simulink model "B3333"  (R2016a)
settings: Solver=FixedStepDiscrete  StartTime=0.0  StopTime=inf  RelTol=1e-3
undefined symbols (not defined in the file): DiscIntNeverNeededParam, Green, led0, Rec, SDTV
libraries: embdlinuxlib x13, visionconversions x8
settings Model: SimulationMode=external  ExtModeTrigDuration=100  Creator=The MathWorks, Inc.  LastModifiedBy=Yewly
settings SolverCC: PositivePriorityOrder=on
settings DataIOCC: LimitDataPoints=on  SaveFormat=Array
settings OptimizationCC: ExpressionDepthLimit=2147483647  OptimizeModelRefInitCode=on  LifeSpan=Inf  MaxStackSize=64
settings DebuggingCC: UnderspecifiedInitializationDetection=Classic  MergeDetectMultiDrivingBlocksExec=none  MultiTaskRateTransMsg=warning  FcnCallInpInsideContextMsg=EnableAllAsWarning  AllowSymbolicDim=off  StateNameClashWarn=warning
settings HardwareCC: ProdBitPerPointer=32  ProdLargestAtomicInteger=Long  ProdLargestAtomicFloat=Double  ProdWordSize=32  ProdHWDeviceType=ARM Compatible->ARM Cortex  UseEmbeddedCoderFeatures=off  UseSimulinkCoderFeatures=off
settings ModelReferenceCC: PropagateSignalLabelsOutOfModel=off
settings RTWCC: SystemTargetFile=ert.tlc  HardwareBoard=Raspberry Pi  TemplateMakefile=ert_default_tmf  GenerateReport=on  RTWVerbose=off  Toolchain=GNU GCC Raspberry Pi  LaunchReport=on
settings CodeAppCC: ForceParamTrailComments=on  IgnoreCustomStorageClasses=off  OperatorAnnotations=on  SimulinkDataObjDesc=on  SFDataObjDesc=on  MATLABFcnDesc=on  MangleLength=10  CustomSymbolStrType=$N$R$M  InsertBlockDesc=on  MATLABSourceComments=on  InternalIdentifier=Classic
settings ERTTargetCC: SupportNonInlinedSFcns=on
settings ConfigComp: CovModelRefEnable=Off

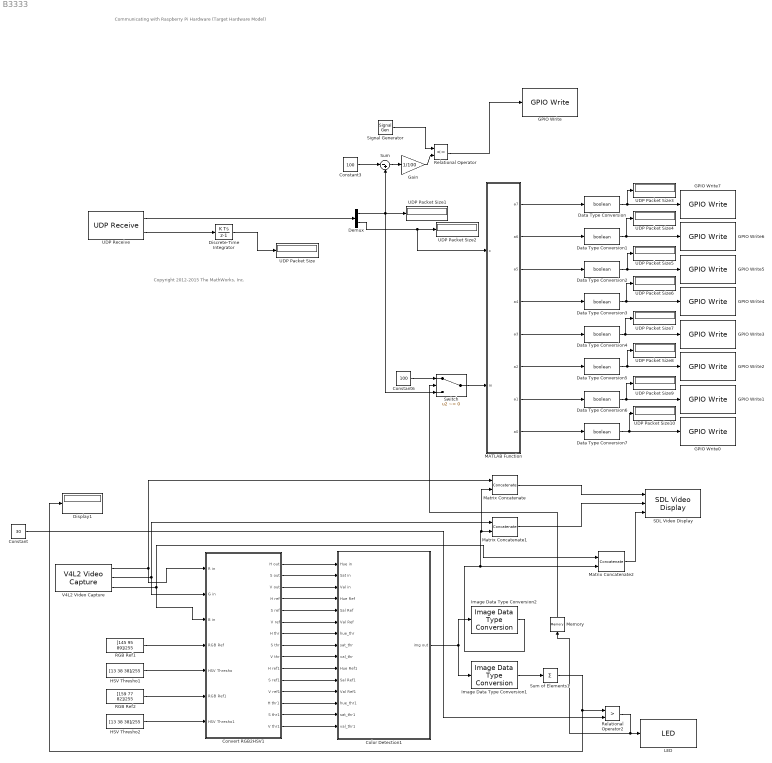
== system B3333 ==
  note: Communicating with Raspberry Pi Hardware
      | (Target Hardware Model)
  note: Copyright 2012-2015 The MathWorks, Inc.
  Color Detection1 : Subsystem
  Constant : Constant  Value=30
  Constant3 : Constant  Value=100
  Constant6 : Constant  Value=100
  Convert RGB2HSV1 : Subsystem
  Data Type Conversion{,1..7} (8 alike) : DataTypeConversion  OutDataTypeStr=boolean
  Demux : Demux  Outputs=2
  Discrete-Time Integrator : DiscreteIntegrator  gainval=1e4  SampleTime=-1  ICPrevOutput=DiscIntNeverNeededParam  ICPrevScaledInput=DiscIntNeverNeededParam
  Display1 : Display
  GPIO Write : embdlinuxlib/GPIO Write  board=Pi 3 Model B  gpio=17  direction=Output  blockPlatform=Raspberry Pi
  GPIO Write0 : embdlinuxlib/GPIO Write  board=Pi 3 Model B  gpio=18  direction=Output  blockPlatform=Raspberry Pi
  GPIO Write1 : embdlinuxlib/GPIO Write  board=Pi 3 Model B  gpio=23  direction=Output  blockPlatform=Raspberry Pi
  GPIO Write2 : embdlinuxlib/GPIO Write  board=Pi 3 Model B  gpio=24  direction=Output  blockPlatform=Raspberry Pi
  GPIO Write3 : embdlinuxlib/GPIO Write  board=Pi 3 Model B  gpio=25  direction=Output  blockPlatform=Raspberry Pi
  GPIO Write4 : embdlinuxlib/GPIO Write  board=Pi 3 Model B  gpio=8  direction=Output  blockPlatform=Raspberry Pi
  GPIO Write5 : embdlinuxlib/GPIO Write  board=Pi 3 Model B  gpio=7  direction=Output  blockPlatform=Raspberry Pi
  GPIO Write6 : embdlinuxlib/GPIO Write  board=Pi 3 Model B  gpio=12  direction=Output  blockPlatform=Raspberry Pi
  "GPIO Write7 " : embdlinuxlib/GPIO Write  board=Pi 3 Model B  gpio=16  direction=Output  blockPlatform=Raspberry Pi
  Gain : Gain  Gain=1/100
  HSV Thresho1 : Constant  Value=[13 38 38]/255
  HSV Thresho2 : Constant  Value=[13 38 38]/255
  Image Data Type Conversion1 : visionconversions/Image Data Type Conversion  outDT=double  isSigned=on  wordLen=16  numFracBits=0
  Image Data Type Conversion2 : visionconversions/Image Data Type Conversion  outDT=uint8  isSigned=on  wordLen=16  numFracBits=0
  LED : embdlinuxlib/LED  board=Model B+  led=led0 (Green)  blockPlatform=Raspberry Pi
  MATLAB Function : MATLAB Function  TreatAsAtomicUnit=on
  Matrix Concatenate : Concatenate  Mode=Multidimensional array  ConcatenateDimension=2
  Matrix Concatenate1 : Concatenate  Mode=Multidimensional array  ConcatenateDimension=2
  Matrix Concatenate2 : Concatenate  Mode=Multidimensional array  ConcatenateDimension=2
  Memory : Memory
  RGB Ref1 : Constant  Value=[145 95 89]/255
  RGB Ref2 : Constant  Value=[159 77 82]/255
  Relational Operator : RelationalOperator  Operator=<=  OutDataTypeStr=boolean
  Relational Operator2 : RelationalOperator  Operator=>  OutDataTypeStr=boolean
  SDL Video Display : embdlinuxlib/SDL Video Display  pixelFormat=RGB  pixelOrder=Planar  rowMajor=on  blockPlatform=Raspberry Pi
  Signal Generator : SignalGenerator  WaveForm=sawtooth  Frequency=200
  Sum : Sum  Inputs=|-+
  Sum of Elements1 : Sum  Inputs=+
  Switch : Switch  Criteria=u2 ~= 0  Threshold=250
  UDP Packet Size{,1..10} (11 alike) : Display
  UDP Receive : embdlinuxlib/UDP Receive  localURL='0.0.0.0'  localPort=25001  remoteURL='0.0.0.0'  remotePort=-1  recvBufferSize=8192  signalDatatype=uint8  dims=2  isVarSize=off  showBlockingTime=off  blockingTime=0  sampletime=1/10000  blockPlatform=Raspberry Pi
  V4L2 Video Capture : embdlinuxlib/V4L2 Video Capture  m_devName='/dev/video0'  roi=[0, 0, 640, 480]  imSizeSelection=Custom  imSize=[80 60]  pixelFormat=RGB  pixelOrder=Planar  sampleTime=1/50  simOutput=Colorbars  blockPlatform=Raspberry Pi
  wires:
  UDP Receive/2 -> Discrete-Time Integrator/1
  Discrete-Time Integrator/1 -> UDP Packet Size/1
  UDP Receive/1 -> Demux/1
  Relational Operator/1 -> GPIO Write/1
  Signal Generator/1 -> Relational Operator/1
  Demux/1 -> Switch/3, Sum/2, UDP Packet Size1/1
  Constant3/1 -> Sum/1
  Sum/1 -> Gain/1
  Gain/1 -> Relational Operator/2
  MATLAB Function/1(a7) -> Data Type Conversion/1
  Data Type Conversion/1 -> UDP Packet Size3/1, "GPIO Write7 "/1
  MATLAB Function/2(a6) -> Data Type Conversion1/1
  Data Type Conversion1/1 -> UDP Packet Size4/1, GPIO Write6/1
  MATLAB Function/3(a5) -> Data Type Conversion2/1
  Data Type Conversion2/1 -> UDP Packet Size5/1, GPIO Write5/1
  MATLAB Function/4(a4) -> Data Type Conversion3/1
  Data Type Conversion3/1 -> GPIO Write4/1, UDP Packet Size6/1
  MATLAB Function/5(a3) -> Data Type Conversion4/1
  Data Type Conversion4/1 -> UDP Packet Size7/1, GPIO Write3/1
  MATLAB Function/6(a2) -> Data Type Conversion5/1
  Data Type Conversion5/1 -> UDP Packet Size8/1, GPIO Write2/1
  MATLAB Function/7(a1) -> Data Type Conversion6/1
  Data Type Conversion6/1 -> UDP Packet Size9/1, GPIO Write1/1
  MATLAB Function/8(a0) -> Data Type Conversion7/1
  Data Type Conversion7/1 -> UDP Packet Size10/1, GPIO Write0/1
  Demux/2 -> MATLAB Function/1(x), UDP Packet Size2/1
  Switch/1 -> MATLAB Function/2(m)
  Constant6/1 -> Switch/1
  Constant/1 -> Relational Operator2/2
  Relational Operator2/1 -> Memory/1, LED/1
  Color Detection1/1(img out) -> Image Data Type Conversion1/1, Image Data Type Conversion2/1
  Sum of Elements1/1 -> Relational Operator2/1, Display1/1
  Image Data Type Conversion2/1 -> Matrix Concatenate/2, Matrix Concatenate1/2, Matrix Concatenate2/2
  Image Data Type Conversion1/1 -> Sum of Elements1/1
  HSV Thresho1/1 -> Convert RGB2HSV1/5(HSV Thresho)
  Convert RGB2HSV1/2(S out) -> Color Detection1/2(Sat in)
  Convert RGB2HSV1/9(V thr) -> Color Detection1/9(val_thr)
  Convert RGB2HSV1/6(V ref) -> Color Detection1/6(Val Ref)
  Convert RGB2HSV1/3(V out) -> Color Detection1/3("Val in ")
  Convert RGB2HSV1/8(S thr) -> Color Detection1/8(sat_thr)
  Convert RGB2HSV1/1(H out) -> Color Detection1/1("Hue in ")
  Convert RGB2HSV1/4(H ref) -> Color Detection1/4(Hue Ref)
  Convert RGB2HSV1/5(S ref) -> Color Detection1/5(Sal Ref)
  Convert RGB2HSV1/7(H thr) -> Color Detection1/7(hue_thr)
  V4L2 Video Capture/1 -> Matrix Concatenate/1, Convert RGB2HSV1/1(R in)
  V4L2 Video Capture/2 -> Matrix Concatenate1/1, Convert RGB2HSV1/2(G in)
  V4L2 Video Capture/3 -> Matrix Concatenate2/1, Convert RGB2HSV1/3(B in)
  RGB Ref1/1 -> Convert RGB2HSV1/4(RGB Ref)
  Convert RGB2HSV1/10(H ref1) -> Color Detection1/10(Hue Ref1)
  Convert RGB2HSV1/11(S ref1) -> Color Detection1/11(Sal Ref1)
  Convert RGB2HSV1/12(V ref1) -> Color Detection1/12(Val Ref1)
  Convert RGB2HSV1/13(H thr1) -> Color Detection1/13(hue_thr1)
  Convert RGB2HSV1/14(S thr1) -> Color Detection1/14(sat_thr1)
  Convert RGB2HSV1/15(V thr1) -> Color Detection1/15(val_thr1)
  HSV Thresho2/1 -> Convert RGB2HSV1/7(HSV Thresho1)
  RGB Ref2/1 -> Convert RGB2HSV1/6(RGB Ref1)
  Matrix Concatenate/1 -> SDL Video Display/1
  Matrix Concatenate1/1 -> SDL Video Display/2
  Matrix Concatenate2/1 -> SDL Video Display/3
  Memory/1 -> Switch/2

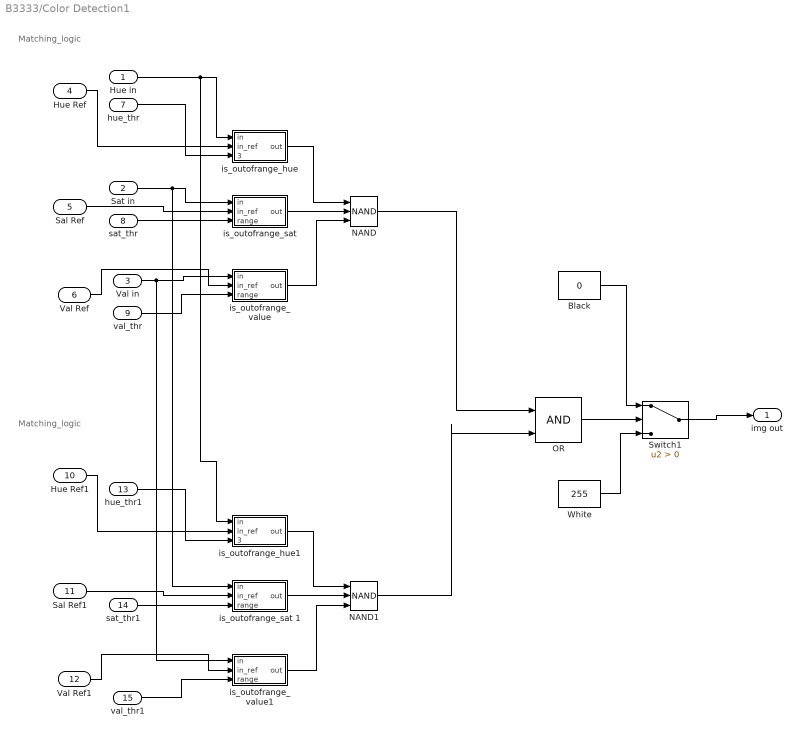
== system B3333/Color Detection1 ==
  note: Matching_logic
  note: Matching_logic
  "Hue in " : Inport
  Sat in : Inport  Port=2
  "Val in " : Inport  Port=3
  Hue Ref : Inport  Port=4
  Sal Ref : Inport  Port=5
  Val Ref : Inport  Port=6
  hue_thr : Inport  Port=7
  sat_thr : Inport  Port=8
  val_thr : Inport  Port=9
  Hue Ref1 : Inport  Port=10
  Sal Ref1 : Inport  Port=11
  Val Ref1 : Inport  Port=12
  hue_thr1 : Inport  Port=13
  sat_thr1 : Inport  Port=14
  val_thr1 : Inport  Port=15
  Black : Constant  Value=0
  NAND : Logic  Operator=NAND  Inputs=3  IconShape=distinctive  AllPortsSameDT=off  OutDataTypeStr=boolean
  NAND1 : Logic  Operator=NAND  Inputs=3  IconShape=distinctive  AllPortsSameDT=off  OutDataTypeStr=boolean
  OR : Logic  IconShape=distinctive  AllPortsSameDT=off  OutDataTypeStr=boolean
  Switch1 : Switch  Criteria=u2 > Threshold  OutDataTypeStr=uint8
  White : Constant  Value=255
  is_outofrange_hue : Subsystem
  is_outofrange_hue1 : Subsystem
  "is_outofrange_sat " : Subsystem
  is_outofrange_sat 1 : Subsystem
  is_outofrange_value : Subsystem
  is_outofrange_value1 : Subsystem
  img out : Outport
  wires:
  is_outofrange_value/1(out) -> NAND/3
  is_outofrange_hue/1(out) -> NAND/1
  Val Ref/1 -> is_outofrange_value/2(in_ref)
  Hue Ref/1 -> is_outofrange_hue/2(in_ref)
  "is_outofrange_sat "/1(out) -> NAND/2
  Sal Ref/1 -> "is_outofrange_sat "/2(in_ref)
  Black/1 -> Switch1/1
  White/1 -> Switch1/3
  hue_thr/1 -> is_outofrange_hue/3("threshold ")
  sat_thr/1 -> "is_outofrange_sat "/3("range ")
  val_thr/1 -> is_outofrange_value/3("range ")
  Switch1/1 -> img out/1
  is_outofrange_value1/1(out) -> NAND1/3
  is_outofrange_hue1/1(out) -> NAND1/1
  "Val in "/1 -> is_outofrange_value1/1(in), is_outofrange_value/1(in)
  Val Ref1/1 -> is_outofrange_value1/2(in_ref)
  Hue Ref1/1 -> is_outofrange_hue1/2(in_ref)
  "Hue in "/1 -> is_outofrange_hue1/1(in), is_outofrange_hue/1(in)
  is_outofrange_sat 1/1(out) -> NAND1/2
  Sal Ref1/1 -> is_outofrange_sat 1/2(in_ref)
  Sat in/1 -> "is_outofrange_sat "/1(in), is_outofrange_sat 1/1(in)
  NAND1/1 -> OR/2
  hue_thr1/1 -> is_outofrange_hue1/3("threshold ")
  sat_thr1/1 -> is_outofrange_sat 1/3("range ")
  val_thr1/1 -> is_outofrange_value1/3("range ")
  NAND/1 -> OR/1
  OR/1 -> Switch1/2

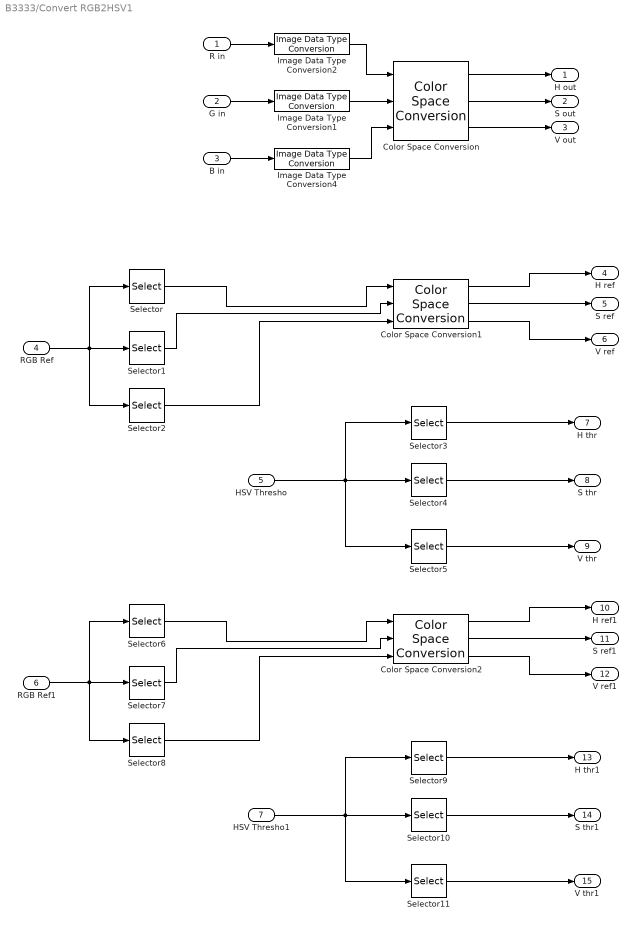
== system B3333/Convert RGB2HSV1 ==
  R in : Inport
  G in : Inport  Port=2
  B in : Inport  Port=3
  RGB Ref : Inport  Port=4
  HSV Thresho : Inport  Port=5
  RGB Ref1 : Inport  Port=6
  HSV Thresho1 : Inport  Port=7
  Color Space Conversion : visionconversions/Color Space  Conversion  conversion=Obsolete  conversionActive=R'G'B' to HSV  wp_str=D65  rec=Rec. 601 (SDTV)  sys=1125/60/2:1  imagePorts=Separate color signals
  Color Space Conversion1 : visionconversions/Color Space  Conversion  conversion=Obsolete  conversionActive=R'G'B' to HSV  wp_str=D65  rec=Rec. 601 (SDTV)  sys=1125/60/2:1  imagePorts=Separate color signals
  Color Space Conversion2 : visionconversions/Color Space  Conversion  conversion=Obsolete  conversionActive=R'G'B' to HSV  wp_str=D65  rec=Rec. 601 (SDTV)  sys=1125/60/2:1  imagePorts=Separate color signals
  Image Data Type Conversion1 : visionconversions/Image Data Type Conversion  outDT=double  isSigned=on  wordLen=16  numFracBits=0
  Image Data Type Conversion2 : visionconversions/Image Data Type Conversion  outDT=double  isSigned=on  wordLen=16  numFracBits=0
  Image Data Type Conversion4 : visionconversions/Image Data Type Conversion  outDT=double  isSigned=on  wordLen=16  numFracBits=0
  Selector{,3,6,9} (4 alike) : Selector  InputPortWidth=3  IndexOptions=Index vector (dialog)  Indices=1  OutputSizes=1
  Selector{1,4,7,10} (4 alike) : Selector  InputPortWidth=3  IndexOptions=Index vector (dialog)  Indices=2  OutputSizes=1
  Selector{2,5,8,11} (4 alike) : Selector  InputPortWidth=3  IndexOptions=Index vector (dialog)  Indices=3  OutputSizes=1
  H out : Outport
  S out : Outport  Port=2
  V out : Outport  Port=3
  H ref : Outport  Port=4
  S ref : Outport  Port=5
  V ref : Outport  Port=6
  H thr : Outport  Port=7
  S thr : Outport  Port=8
  V thr : Outport  Port=9
  H ref1 : Outport  Port=10
  S ref1 : Outport  Port=11
  V ref1 : Outport  Port=12
  H thr1 : Outport  Port=13
  S thr1 : Outport  Port=14
  V thr1 : Outport  Port=15
  wires:
  Color Space Conversion/2 -> S out/1
  Image Data Type Conversion1/1 -> Color Space Conversion/2
  R in/1 -> Image Data Type Conversion2/1
  G in/1 -> Image Data Type Conversion1/1
  Color Space Conversion1/3 -> V ref/1
  Selector1/1 -> Color Space Conversion1/2
  Selector4/1 -> S thr/1
  Selector5/1 -> V thr/1
  Color Space Conversion/3 -> V out/1
  Selector2/1 -> Color Space Conversion1/3
  Selector3/1 -> H thr/1
  Image Data Type Conversion2/1 -> Color Space Conversion/1
  Color Space Conversion1/1 -> H ref/1
  Color Space Conversion/1 -> H out/1
  Image Data Type Conversion4/1 -> Color Space Conversion/3
  Color Space Conversion1/2 -> S ref/1
  Selector/1 -> Color Space Conversion1/1
  B in/1 -> Image Data Type Conversion4/1
  HSV Thresho/1 -> Selector3/1, Selector5/1, Selector4/1
  RGB Ref/1 -> Selector2/1, Selector1/1, Selector/1
  Color Space Conversion2/3 -> V ref1/1
  Selector7/1 -> Color Space Conversion2/2
  Selector10/1 -> S thr1/1
  Selector11/1 -> V thr1/1
  Selector8/1 -> Color Space Conversion2/3
  Selector9/1 -> H thr1/1
  Color Space Conversion2/1 -> H ref1/1
  Color Space Conversion2/2 -> S ref1/1
  Selector6/1 -> Color Space Conversion2/1
  HSV Thresho1/1 -> Selector9/1, Selector11/1, Selector10/1
  RGB Ref1/1 -> Selector8/1, Selector7/1, Selector6/1

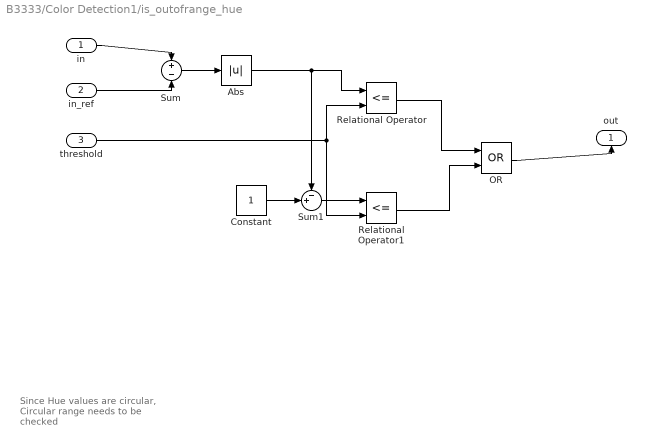
== system B3333/Color Detection1/is_outofrange_hue ==
  note: Since Hue values are circular, Circular range needs to be checked
  in : Inport
  in_ref : Inport  Port=2
  "threshold " : Inport  Port=3
  Abs : Abs
  Constant : Constant
  "OR " : Logic  Operator=OR  AllPortsSameDT=off  OutDataTypeStr=boolean
  Relational Operator : RelationalOperator  Operator=<=  OutDataTypeStr=boolean
  Relational Operator1 : RelationalOperator  Operator=<=  OutDataTypeStr=boolean
  Sum : Sum  Inputs=+|-
  Sum1 : Sum  Inputs=-+|
  out : Outport
  wires:
  in/1 -> Sum/1
  in_ref/1 -> Sum/2
  Sum/1 -> Abs/1
  Abs/1 -> Sum1/1, Relational Operator/1
  "threshold "/1 -> Relational Operator1/2, Relational Operator/2
  Constant/1 -> Sum1/2
  Sum1/1 -> Relational Operator1/1
  Relational Operator/1 -> "OR "/1
  Relational Operator1/1 -> "OR "/2
  "OR "/1 -> out/1

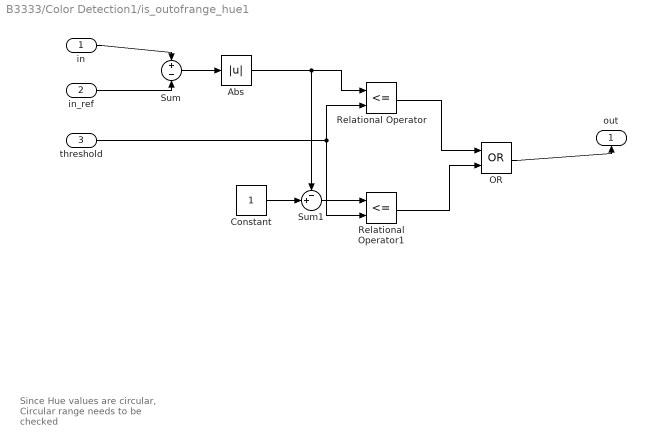
== system B3333/Color Detection1/is_outofrange_hue1 ==
  note: Since Hue values are circular, Circular range needs to be checked
  in : Inport
  in_ref : Inport  Port=2
  "threshold " : Inport  Port=3
  Abs : Abs
  Constant : Constant
  "OR " : Logic  Operator=OR  AllPortsSameDT=off  OutDataTypeStr=boolean
  Relational Operator : RelationalOperator  Operator=<=  OutDataTypeStr=boolean
  Relational Operator1 : RelationalOperator  Operator=<=  OutDataTypeStr=boolean
  Sum : Sum  Inputs=+|-
  Sum1 : Sum  Inputs=-+|
  out : Outport
  wires:
  in/1 -> Sum/1
  in_ref/1 -> Sum/2
  Sum/1 -> Abs/1
  Abs/1 -> Sum1/1, Relational Operator/1
  "threshold "/1 -> Relational Operator1/2, Relational Operator/2
  Constant/1 -> Sum1/2
  Sum1/1 -> Relational Operator1/1
  Relational Operator/1 -> "OR "/1
  Relational Operator1/1 -> "OR "/2
  "OR "/1 -> out/1

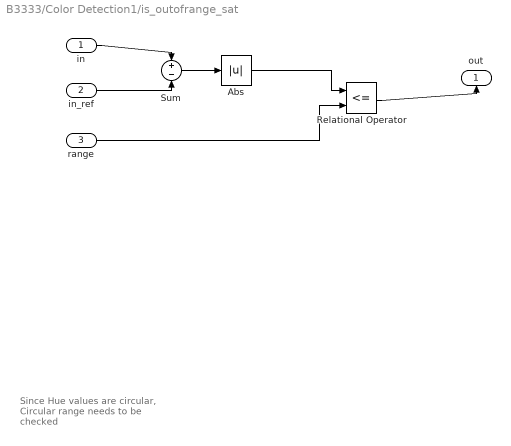
== system B3333/Color Detection1/is_outofrange_sat  ==
  note: Since Hue values are circular, Circular range needs to be checked
  in : Inport
  in_ref : Inport  Port=2
  "range " : Inport  Port=3
  Abs : Abs
  Relational Operator : RelationalOperator  Operator=<=  OutDataTypeStr=boolean
  Sum : Sum  Inputs=+|-
  out : Outport
  wires:
  in/1 -> Sum/1
  in_ref/1 -> Sum/2
  Sum/1 -> Abs/1
  Abs/1 -> Relational Operator/1
  "range "/1 -> Relational Operator/2
  Relational Operator/1 -> out/1

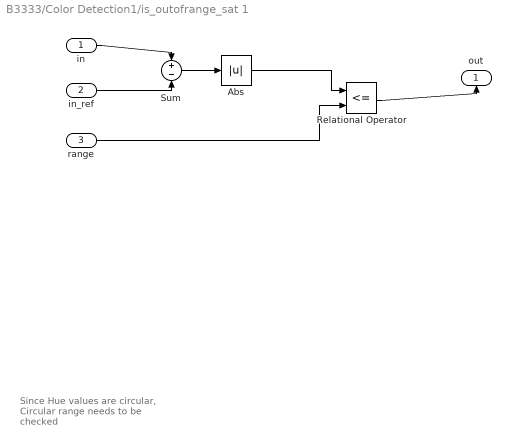
== system B3333/Color Detection1/is_outofrange_sat 1 ==
  note: Since Hue values are circular, Circular range needs to be checked
  in : Inport
  in_ref : Inport  Port=2
  "range " : Inport  Port=3
  Abs : Abs
  Relational Operator : RelationalOperator  Operator=<=  OutDataTypeStr=boolean
  Sum : Sum  Inputs=+|-
  out : Outport
  wires:
  in/1 -> Sum/1
  in_ref/1 -> Sum/2
  Sum/1 -> Abs/1
  Abs/1 -> Relational Operator/1
  "range "/1 -> Relational Operator/2
  Relational Operator/1 -> out/1

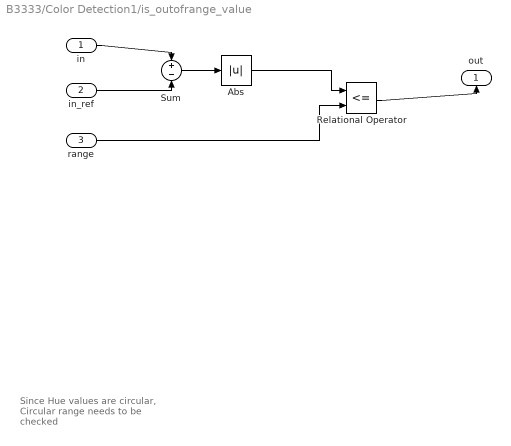
== system B3333/Color Detection1/is_outofrange_value ==
  note: Since Hue values are circular, Circular range needs to be checked
  in : Inport
  in_ref : Inport  Port=2
  "range " : Inport  Port=3
  Abs : Abs
  Relational Operator : RelationalOperator  Operator=<=  OutDataTypeStr=boolean
  Sum : Sum  Inputs=+|-
  out : Outport
  wires:
  in/1 -> Sum/1
  in_ref/1 -> Sum/2
  Sum/1 -> Abs/1
  Abs/1 -> Relational Operator/1
  "range "/1 -> Relational Operator/2
  Relational Operator/1 -> out/1

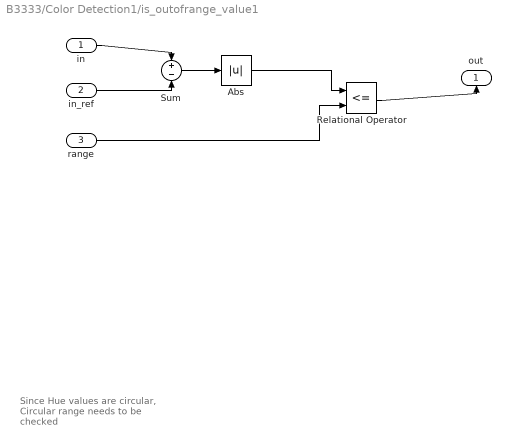
== system B3333/Color Detection1/is_outofrange_value1 ==
  note: Since Hue values are circular, Circular range needs to be checked
  in : Inport
  in_ref : Inport  Port=2
  "range " : Inport  Port=3
  Abs : Abs
  Relational Operator : RelationalOperator  Operator=<=  OutDataTypeStr=boolean
  Sum : Sum  Inputs=+|-
  out : Outport
  wires:
  in/1 -> Sum/1
  in_ref/1 -> Sum/2
  Sum/1 -> Abs/1
  Abs/1 -> Relational Operator/1
  "range "/1 -> Relational Operator/2
  Relational Operator/1 -> out/1

== matlab function B3333/MATLAB Function ==
  data: x input; a7 output; a6 output; a5 output; a4 output; a3 output; a2 output; a1 output; a0 output; m input
function [a7,a6,a5,a4,a3,a2,a1,a0]= fcn(x,m)
%#codegen
y = [0 0 0 0 0 0 0 0];
u = x;
if(u > 127)
    y(8) = 1;
    u = u - (128);
else
    y(8) = 0;
end


if(u > 63)
    y(7) = 1;
    u = u - (64);
else
    y(7) = 0;
end

if(u > 31)
    y(6) = 1;
    u = u - (32);
else
    y(6) = 0;
end

if(u > 15)
    y(5) = 1;
    u = u - (16);
else
    y(5) = 0;
end

if(u > 7)
    y(4) = 1;
    u = u - (8);
else
    y(4) = 0;
end

if(u > 3)
    y(3) = 1;
    u = u - (4);
else
    y(3) = 0;
end

if(u > 1)
    y(2) = 1;
    u = u - (2);
else
    y(2) = 0;
end

if(u > 0)
    y(1) = 1;
else
    y(1) = 0;
end
if(m==100)
    y(2) = 1;
else
    y(2) = 0;
end
a7 = y(8);
a6 = y(7);
a5 = y(6);
a4 = y(5);
a3 = y(4);
a2 = y(3);
a1 = y(2);
a0 = 0;
